simulink model "assignmentblock"  (R2021a)
settings: Solver=VariableStepAuto  StartTime=0.0  StopTime=10.0  RelTol=1e-3
settings Model: Creator=surya  LastModifiedBy=surya

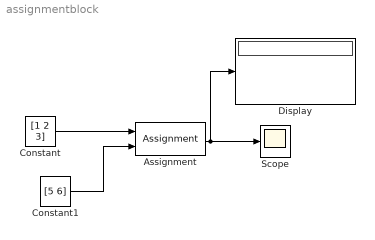
== system assignmentblock ==
  Assignment : Assignment  DiagnosticForDimensions=Warning  IndexOptions=Index vector (dialog)  Indices=[1 2]  OutputSizes=1
  Constant : Constant  Value=[1 2 3]
  Constant1 : Constant  Value=[5 6]
  Display : Display
  Scope : Scope
  wires:
  Constant/1 -> Assignment/1
  Constant1/1 -> Assignment/2
  Assignment/1 -> Scope/1, Display/1
